simulink model "TransmissionController"  (R2020a)
settings: Solver=FixedStepDiscrete  StartTime=0.0  StopTime=inf  FixedStep=0.01  RelTol=1e-3  EnableMultiTasking=on
undefined symbols (not defined in the file): Dn_Shft_Spd, Gear_Dn_bpt, Gear_Up_bpt, Pdl_Pos_Dn_bpt, Pdl_Pos_Up_bpt, Up_Shft_Spd
settings Model: DataDictionary=System_Data_Dictionary.sldd  ModifiedByFormat=The MathWorks, Inc.  OrderedModelArguments=off  Creator=The MathWorks, Inc.  LastModifiedBy=The MathWorks, Inc.
settings SolverCC: AutoInsertRateTranBlk=on
settings DataIOCC: SaveOutput=off  SaveTime=off  ReturnWorkspaceOutputs=off
settings OptimizationCC: UseDivisionForNetSlopeComputation=on
settings DebuggingCC: ArithmeticOperatorsInVariantConditions=warning
settings SFSimCC: SimUseLocalCustomCode=off  CustomCodeUndefinedFunction=UseInterfaceOnly
settings RTWCC: RTWUseLocalCustomCode=off
settings CodeAppCC: StateflowObjectComments=on

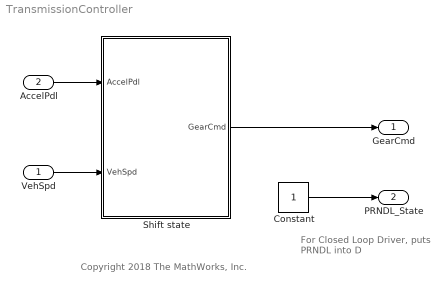
== system TransmissionController ==
  note: For Closed Loop Driver,
      | puts PRNDL into D
  note: Copyright 2018 The MathWorks, Inc.
  VehSpd : Inport
  AccelPdl : Inport  Port=2
  Constant : Constant  SampleTime=0.01
  Shift state : Subsystem
  GearCmd : Outport  VectorParamsAs1DForOutWhenUnconnected=off
  PRNDL_State : Outport  Port=2  VectorParamsAs1DForOutWhenUnconnected=off
  wires:
  AccelPdl/1 -> Shift state/1(AccelPdl)
  VehSpd/1 -> Shift state/2(VehSpd)
  Shift state/1(GearCmd) -> GearCmd/1
  Constant/1 -> PRNDL_State/1

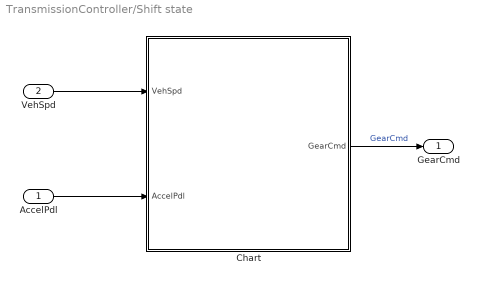
== system TransmissionController/Shift state ==
  AccelPdl : Inport
  VehSpd : Inport  Port=2
  Chart : Stateflow chart  TreatAsAtomicUnit=on
  GearCmd : Outport  VectorParamsAs1DForOutWhenUnconnected=off
  wires:
  AccelPdl/1 -> Chart/2(AccelPdl)
  Chart/1(GearCmd) -> GearCmd/1  "GearCmd"
  VehSpd/1 -> Chart/1(VehSpd)

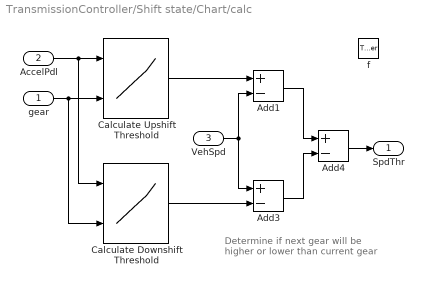
== system TransmissionController/Shift state/Chart/calc ==
  note: Determine if next gear will be
      | higher or lower than current gear
  gear : Inport
  AccelPdl : Inport  Port=2
  VehSpd : Inport  Port=3
  f : TriggerPort  TriggerType=function-call  VariantControl=Variant  StatesWhenEnabling=reset
      settings: CopyFcn=Stateflow.SLINSF.SimulinkMan.removeBlockPreDeleteFcn  PreDeleteFcn=Stateflow.SLINSF.SimulinkMan.unsafePredeleteFcn
  Add1 : Sum  Inputs=+-
  Add3 : Sum  Inputs=+-
  Add4 : Sum  Inputs=+-
  Calculate Upshift Threshold : Lookup_n-D  BreakpointsForDimension1=Pdl_Pos_Up_bpt  BreakpointsForDimension2=Gear_Up_bpt  Table=Up_Shft_Spd  ExtrapMethod=Clip  UseLastTableValue=on  InternalRulePriority=Speed  RndMeth=Simplest  InputSameDT=on
  Calculate Downshift Threshold : Lookup_n-D  BreakpointsForDimension1=Pdl_Pos_Dn_bpt  BreakpointsForDimension2=Gear_Dn_bpt  Table=Dn_Shft_Spd  ExtrapMethod=Clip  UseLastTableValue=on  InternalRulePriority=Speed  RndMeth=Simplest  InputSameDT=on
  SpdThr : Outport  VectorParamsAs1DForOutWhenUnconnected=off
  wires:
  AccelPdl/1 -> Calculate Downshift Threshold/1, Calculate Upshift Threshold/1
  gear/1 -> Calculate Downshift Threshold/2, Calculate Upshift Threshold/2
  Calculate Downshift Threshold/1 -> Add3/2
  Calculate Upshift Threshold/1 -> Add1/1
  VehSpd/1 -> Add1/2, Add3/1
  Add1/1 -> Add4/1
  Add3/1 -> Add4/2
  Add4/1 -> SpdThr/1

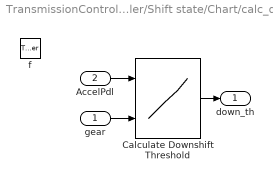
== system TransmissionController/Shift state/Chart/calc_down ==
  gear : Inport
  AccelPdl : Inport  Port=2
  f : TriggerPort  TriggerType=function-call  VariantControl=Variant  StatesWhenEnabling=reset
      settings: CopyFcn=Stateflow.SLINSF.SimulinkMan.removeBlockPreDeleteFcn  PreDeleteFcn=Stateflow.SLINSF.SimulinkMan.unsafePredeleteFcn
  Calculate Downshift Threshold : Lookup_n-D  BreakpointsForDimension1=Pdl_Pos_Dn_bpt  BreakpointsForDimension2=Gear_Dn_bpt  Table=Dn_Shft_Spd  ExtrapMethod=Clip  UseLastTableValue=on  InternalRulePriority=Speed  RndMeth=Simplest  InputSameDT=on
  down_th : Outport  VectorParamsAs1DForOutWhenUnconnected=off
  wires:
  Calculate Downshift Threshold/1 -> down_th/1
  gear/1 -> Calculate Downshift Threshold/2
  AccelPdl/1 -> Calculate Downshift Threshold/1

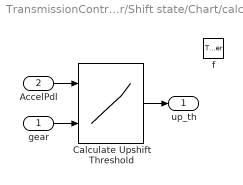
== system TransmissionController/Shift state/Chart/calc_up ==
  gear : Inport
  AccelPdl : Inport  Port=2
  f : TriggerPort  TriggerType=function-call  VariantControl=Variant  StatesWhenEnabling=reset
      settings: CopyFcn=Stateflow.SLINSF.SimulinkMan.removeBlockPreDeleteFcn  PreDeleteFcn=Stateflow.SLINSF.SimulinkMan.unsafePredeleteFcn
  Calculate Upshift Threshold : Lookup_n-D  BreakpointsForDimension1=Pdl_Pos_Up_bpt  BreakpointsForDimension2=Gear_Up_bpt  Table=Up_Shft_Spd  ExtrapMethod=Clip  UseLastTableValue=on  InternalRulePriority=Speed  RndMeth=Simplest  InputSameDT=on
  up_th : Outport  VectorParamsAs1DForOutWhenUnconnected=off
  wires:
  Calculate Upshift Threshold/1 -> up_th/1
  AccelPdl/1 -> Calculate Upshift Threshold/1
  gear/1 -> Calculate Upshift Threshold/2

== stateflow chart TransmissionController/Shift state/Chart ==
  settings: sampleTime=0.01  enableNonTerminalStates=1
  state GearCmd [parallel]
    settings: executionOrder=1
    state G1
      en:
      GearCmd = 1;
    state G2
      en:
      GearCmd = 2;
      du:
      [SpdThr] = calc(2,AccelPdl,VehSpd);
    state G3
      en:
      GearCmd = 3;
      du:
      [SpdThr] = calc(3,AccelPdl,VehSpd);
    state G6
      en:
      GearCmd = 6;
    state G5
      en:
      GearCmd = 5;
      du:
      [SpdThr] = calc(5,AccelPdl,VehSpd);
    state G4
      en:
      GearCmd = 4;
      du:
      [SpdThr] = calc(4,AccelPdl,VehSpd);
    (default) -> G1
    G1 -> G2 : Up
    G2 -> G3 [order 1] : Up
    G2 -> G1 [order 2] : Down
    G3 -> G2 [order 2] : Down
    G3 -> G4 [order 1] : Up
    G4 -> G3 [order 2] : Down
    G5 -> G6 [order 1] : Up
    G4 -> G5 [order 1] : Up
    G5 -> G4 [order 2] : Down
    G6 -> G5 : Down
  state SelectionState [parallel]
    du:[up_th]=calc_up(GearCmd,AccelPdl);
    du:[down_th]=calc_down(GearCmd,AccelPdl);
    settings: executionOrder=2
    state SteadyState
      en:
      clutchControl = 0;
    state preDownShifting
    state preUpShifting
    state DownShifting
      en:
      GearCmd = GearCmd - 0.5;
    state UpShifting
      en:
      GearCmd = GearCmd + 0.5;
    (default) -> SteadyState
    SteadyState -> (junction 62) [order 1] : [VehSpd < down_th && ...
        | GearCmd > 1]
    SteadyState -> (junction 128) [order 2] : [VehSpd > up_th &&...
        | GearCmd <= 5 && ...
        | floor(GearCmd) == GearCmd]
    (junction 62) -> preDownShifting
    (junction 128) -> preUpShifting
    (junction 168) -> SteadyState
    (junction 23) -> SteadyState
    (junction 161) -> SteadyState
    preDownShifting -> (junction 168) [order 2] : [VehSpd >= down_th]
    preUpShifting -> (junction 161) [order 2] : [VehSpd <= up_th]
    preDownShifting -> DownShifting [order 1] : after(0.5, sec)
        | [VehSpd < down_th]
    preUpShifting -> UpShifting [order 1] : after(0.5,sec)
        | [VehSpd > up_th]
    DownShifting -> (junction 23) : {GearCmd.Down;}
    UpShifting -> (junction 23) : {GearCmd.Up;}
  state up_th = calc_up(gear,AccelPdl) [function]
  state down_th = calc_down(gear,AccelPdl) [function]
  state SpdThr = calc(gear,AccelPdl,VehSpd) [function]
  data: gear function_input; AccelPdl function_input; up_th function_output; gear function_input; AccelPdl function_input; down_th function_output; gear function_input; AccelPdl function_input; SpdThr function_output; VehSpd function_input; GearCmd output double =1; VehSpd input; AccelPdl input; clutchControl local double; SpdThr local double; up_th local double; down_th local double
  events: Up local EITHER_EDGE_EVENT; Down local EITHER_EDGE_EVENT
